simulink model "model_conti_input"  (R2014b)
settings: Solver=ode45  StartTime=0.0  StopTime=10.0  RelTol=1e-3
values from neighbouring files (symbols this model uses):
  A = [0 0 1 0; 0 0 0 1; -3 1 -0.4 0.1; 1 -1 0.1 -0.1]    [HW7_main.m]
  B = [0 0; 0 0; 1 0; 0 1]    [HW7_main.m]
  C = [1 0 0 0; 0 1 0 0]    [HW7_main.m]
  Ec = -inv(Rc)*B'*inv(A - B*Kc)'*C'*Qc    [HW7_main.m]
  Ko = Ko'    [HW7_main.m]
  Tf = 5e-5    (= 5e-05)    [HW7_main.m]
  x_ini = [0.3 -0.2 -0.1 0.2]'    [HW7_main.m]
undefined symbols (not defined in the file or in its folder): Kc
settings Model: Creator=123  LastModifiedBy=123

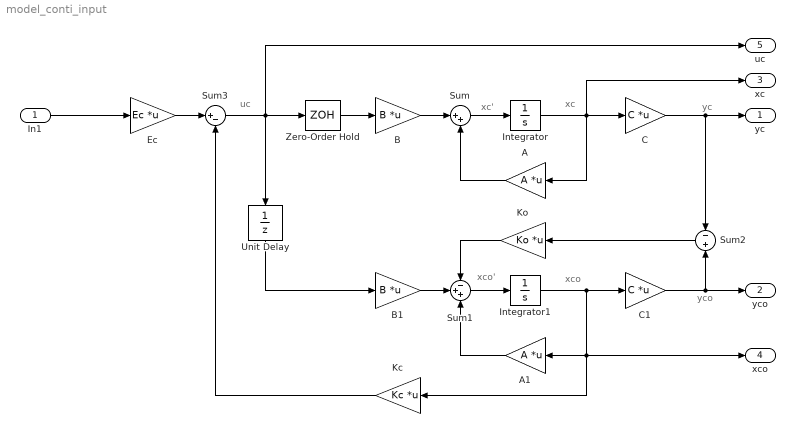
== system model_conti_input ==
  note: uc
  note: yco
  note: yc
  note: xc
  note: xc'
  note: xco
  note: xco'
  In1 : Inport
  A : Gain  Gain=A  Multiplication=Matrix(K*u)
  A1 : Gain  Gain=A  Multiplication=Matrix(K*u)
  B : Gain  Gain=B  Multiplication=Matrix(K*u)
  B1 : Gain  Gain=B  Multiplication=Matrix(K*u)
  C : Gain  Gain=C  Multiplication=Matrix(K*u)
  C1 : Gain  Gain=C  Multiplication=Matrix(K*u)
  Ec : Gain  Gain=Ec  Multiplication=Matrix(K*u)
  Integrator : Integrator  InitialCondition=x_ini
  Integrator1 : Integrator  InitialCondition=pinv(C)*(C*x_ini)
  Kc : Gain  Gain=Kc  Multiplication=Matrix(K*u)
  Ko : Gain  Gain=Ko  Multiplication=Matrix(K*u)
  Sum : Sum  Inputs=|++
  Sum1 : Sum  Inputs=-++
  Sum2 : Sum  Inputs=-|+
  Sum3 : Sum  Inputs=|+-
  Unit Delay : UnitDelay  SampleTime=Tf
  Zero-Order Hold : ZeroOrderHold  SampleTime=Tf
  yc : Outport
  yco : Outport  Port=2
  xc : Outport  Port=3
  xco : Outport  Port=4
  uc : Outport  Port=5
  wires:
  Integrator/1 -> xc/1, C/1, A/1
  B/1 -> Sum/1
  Sum/1 -> Integrator/1
  A/1 -> Sum/2
  Zero-Order Hold/1 -> B/1
  C/1 -> Sum2/1, yc/1
  Sum1/1 -> Integrator1/1
  Unit Delay/1 -> B1/1
  C1/1 -> Sum2/2, yco/1
  Sum3/1 -> uc/1, Zero-Order Hold/1, Unit Delay/1
  B1/1 -> Sum1/2
  Ko/1 -> Sum1/1
  A1/1 -> Sum1/3
  Sum2/1 -> Ko/1
  Integrator1/1 -> C1/1, xco/1, A1/1, Kc/1
  Ec/1 -> Sum3/1
  In1/1 -> Ec/1
  Kc/1 -> Sum3/2
